simulink model "soccer"  (Simulink 4.00)
settings: Solver=ode45  StartTime=0.0  StopTime=150  RelTol=1e-3
PostLoadFcn:
  | init_motes
InitFcn:
  | clear functions
undefined symbols (not defined in the file or in its folder): WLAN, xBall, xPos, yBall, yPos
libraries: truetime x11
settings Model: Creator=anton  LastModifiedBy=anton  SaveTime=off  SaveOutput=off  RTWOptions="-aEnforceIntegerDowncast=1 -aFoldNonRolledExpr=1 -aInlineInvariantSignals=0 -aInlineParameters=0 -aLocalBlockOutputs=1 -aRollThreshold=5 -aGenerateReport=0 -aGenCodeOnly=0 -aRTWVerbose=1 -aIncludeHyperlinkInReport=0 -aLaunchReport=0 -aForceParamTrailComments=0 -aGenerateComments=1 -aIgnoreCustomStorageClasses=1 -aIncHierarchyInIds=0 -aMaxRTWIdLen=31 -aShowEliminatedStatements=0 -aPrefixModelToSubsysFcnNames=1 -aIncDataTypeInIds=0 -aInsertBlockDesc=0 -aSimulinkBlockComments=1 -aInlinedPrmAccess=\"Literals\"  -aSuppressErrorStatus=0 -aModelReferenceCompliant=1 -aSupportNonInlinedSFcns=1 -aSupportContinuousTime=1 -aSupportComplex=1 -aSupportNonFinite=1 -aSupportAbsoluteTime=1 -aTargetPreCompLibLocation=\"\" -aTargetLibSuffix=\"\" -aTargetFcnLib=\"ansi_tfl_tmw.mat\" -aMultiInstanceERTCode=0 -aLogVarNameModifier=\"rt_\" -aERTFirstTimeCompliant=0 -aIsPILTarget=0 -aCombineOutputUpdateFcns=0 -aGenerateASAP2=0 -aGenerateTestInterfaces=0 -aGenerateSampleERTMain=0 -aGenerateFullHeader=1 -aUtilityFuncGeneration=\"Auto\" -aIncludeFileDelimiter=\"Auto\" -aIncludeERTFirstTime=1 -aIncludeMdlTerminateFcn=1 -aPurelyIntegerCode=0 -aERTCustomFileBanners=0 -aRTWCAPIStates=0 -aRTWCAPIParams=0 -aRTWCAPISignals=0 -aMatFileLogging=1 -aGenFloatMathFcnCalls=\"ANSI_C\" -aExtModeMexFile=\"ext_comm\" -aExtModeTransport=0 -aExtModeStaticAllocSize=1000000 -aExtModeTesting=0 -aExtModeStaticAlloc=0 -aExtMode=0"  ExtModeAutoUpdateStatusClock=off  BlockReductionOpt=off

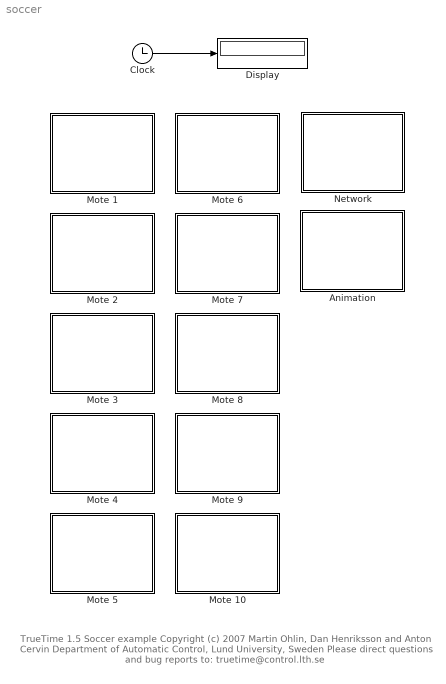
== system soccer ==
  note: TrueTime 1.5  Soccer example
      | Copyright (c) 2007
      | Martin Ohlin, Dan Henriksson and Anton Cervin
      | Department of Automatic Control, Lund University, Sweden
      | Please direct questions and bug reports to:  truetime@control.lth.se
  Animation : Subsystem  mask{N=10}
      mask prompts: N "Number of nodes"
      mask init:
      | %Remove all "From" blocks
      | %Remove all lines from the "From" blocks
      | muxblocks = {'xMux', 'yMux'};
      | fromblocks={'x', 'y'};
      | for j=1:length(muxblocks),
      |   Nold=str2num(get_param(strcat(strcat(gcb,'/'), muxblocks{j}),'Inputs'));
      |   for k=1:Nold
      |     to_name=strcat(strcat(muxblocks{j}, '/'), num2str(k));
      |     from_name=strcat(strcat(fromblocks{j}, num2str(k)), '/1');
      |     delete_line(gcb, from_name, to_name);
      |     delete_block(strcat(strcat(gcb, '/'), strcat(fromblocks{j}, num2str(k))));
      |   end
      |   set_param(strcat(strcat(gcb,'/'), muxblocks{j}),'Inputs',num2str(N));
      | end
      | 
      | for k=1:N
      |     name=strcat(strcat(gcb,'/x'),num2str(k));
      |     add_block('built-in/From',name,'Position',[15 15+(k-1)*20 45 15+k*20],'GotoTag',strcat('x',num2str(k)));
      |     add_line(gcb,strcat(strcat('x',num2str(k)),'/1'),strcat('xMux/',num2str(k)));
      |     
      |     name=strcat(strcat(gcb,'/y'),num2str(k));
      |     add_block('built-in/From',name,'Position',[80 150+(k-1)*20 110 150+k*20],'GotoTag',strcat('y',num2str(k)));
      |     add_line(gcb,strcat(strcat('y',num2str(k)),'/1'),strcat('yMux/',num2str(k)));
      | end
      settings: RTWFcnNameOpts=Auto  RTWFileNameOpts=Auto
  Clock : Clock
      settings: DisplayTime=off  Decimation=10
  Display : Display
      settings: Format=short
  Mote 1 : Subsystem  mask(fgdfgMOTE){nodeID=1}
      mask prompts: nodeID "Node number"
      mask init:
      | set_param(strcat(gcb,'/From_rcv'),'GotoTag',strcat('rcv',num2str(nodeID)));
      | set_param(strcat(gcb,'/Goto_x'),'GotoTag',strcat('x',num2str(nodeID)));
      | set_param(strcat(gcb,'/Goto_y'),'GotoTag',strcat('y',num2str(nodeID)));
      | set_param(strcat(gcb,'/Goto_snd'),'GotoTag',strcat('snd',num2str(nodeID)));
      settings: RTWFcnNameOpts=Auto  RTWFileNameOpts=Auto
  Mote 10 : Subsystem  mask(fgdfgMOTE){nodeID=10}
      mask prompts: nodeID "Node number"
      mask init: same as soccer/Mote 1
      settings: RTWFcnNameOpts=Auto  RTWFileNameOpts=Auto
  Mote 2 : Subsystem  mask(fgdfgMOTE){nodeID=2}
      mask prompts: nodeID "Node number"
      mask init: same as soccer/Mote 1
      settings: RTWFcnNameOpts=Auto  RTWFileNameOpts=Auto
  Mote 3 : Subsystem  mask(fgdfgMOTE){nodeID=3}
      mask prompts: nodeID "Node number"
      mask init: same as soccer/Mote 1
      settings: RTWFcnNameOpts=Auto  RTWFileNameOpts=Auto
  Mote 4 : Subsystem  mask(fgdfgMOTE){nodeID=4}
      mask prompts: nodeID "Node number"
      mask init: same as soccer/Mote 1
      settings: RTWFcnNameOpts=Auto  RTWFileNameOpts=Auto
  Mote 5 : Subsystem  mask(fgdfgMOTE){nodeID=5}
      mask prompts: nodeID "Node number"
      mask init: same as soccer/Mote 1
      settings: RTWFcnNameOpts=Auto  RTWFileNameOpts=Auto
  Mote 6 : Subsystem  mask(fgdfgMOTE){nodeID=6}
      mask prompts: nodeID "Node number"
      mask init: same as soccer/Mote 1
      settings: RTWFcnNameOpts=Auto  RTWFileNameOpts=Auto
  Mote 7 : Subsystem  mask(fgdfgMOTE){nodeID=7}
      mask prompts: nodeID "Node number"
      mask init: same as soccer/Mote 1
      settings: RTWFcnNameOpts=Auto  RTWFileNameOpts=Auto
  Mote 8 : Subsystem  mask(fgdfgMOTE){nodeID=8}
      mask prompts: nodeID "Node number"
      mask init: same as soccer/Mote 1
      settings: RTWFcnNameOpts=Auto  RTWFileNameOpts=Auto
  Mote 9 : Subsystem  mask(fgdfgMOTE){nodeID=9}
      mask prompts: nodeID "Node number"
      mask init: same as soccer/Mote 1
      settings: RTWFcnNameOpts=Auto  RTWFileNameOpts=Auto
  Network : Subsystem  mask{N=10}
      mask prompts: N "Number of nodes"
      mask init:
      | %Remove all "From" blocks
      | %Remove all lines from the "From" blocks
      | muxblocks = {'sndMux', 'xMux', 'yMux'};
      | fromblocks={'snd', 'x', 'y'};
      | for j=1:length(muxblocks),
      |   Nold=str2num(get_param(strcat(strcat(gcb,'/'), muxblocks{j}),'Inputs'));
      |   for k=1:Nold
      |     to_name=strcat(strcat(muxblocks{j}, '/'), num2str(k));
      |     from_name=strcat(strcat(fromblocks{j}, num2str(k)), '/1');
      |     delete_line(gcb, from_name, to_name);
      |     delete_block(strcat(strcat(gcb, '/'), strcat(fromblocks{j}, num2str(k))));
      |   end
      |   set_param(strcat(strcat(gcb,'/'), muxblocks{j}),'Inputs',num2str(N));
      | end
      | 
      | %Remove all "Goto" blocks
      | %Remove all lines to the "Goto" block
      | demuxblocks={'Demux'};
      | gotoblocks={'rcv'};
      | for j=1:length(demuxblocks)
      |   Nold=str2num(get_param(strcat(strcat(gcb,'/'), demuxblocks{j}),'Outputs'));
      |   for k=1:Nold
      |     from_name=strcat(strcat(demuxblocks{j}, '/'), num2str(k));
      |     to_name=strcat(strcat(gotoblocks{j}, num2str(k)), '/1');
      |     delete_line(gcb, from_name, to_name);
      |     delete_block(strcat(strcat(gcb, '/'), strcat(gotoblocks{j}, num2str(k))));
      |   end
      |   set_param(strcat(strcat(gcb, '/'), demuxblocks{j}), 'Outputs',num2str(N));
      | end
      | 
      | 
      | for k=1:N
      |     name=strcat(strcat(gcb,'/snd'),num2str(k));
      |     add_block('built-in/From',name,'Position',[15 30+(k-1)*20 45 30+k*20],'GotoTag',strcat('snd',num2str(k)));
      |     add_line(gcb,strcat(strcat('snd',num2str(k)),'/1'),strcat('sndMux/',num2str(k)));
      |     
      |     name=strcat(strcat(gcb,'/x'),num2str(k));
      |     add_block('built-in/From',name,'Position',[60 130+(k-1)*20 90 130+k*20],'GotoTag',strcat('x',num2str(k)));
      |     add_line(gcb,strcat(strcat('x',num2str(k)),'/1'),strcat('xMux/',num2str(k)));
      |     
      |     name=strcat(strcat(gcb,'/y'),num2str(k));
      |     add_block('built-in/From',name,'Position',[105 230+(k-1)*20 135 230+k*20],'GotoTag',strcat('y',num2str(k)));
      |     add_line(gcb,strcat(strcat('y',num2str(k)),'/1'),strcat('yMux/',num2str(k)));
      | 
      |     name=strcat(strcat(gcb,'/rcv'),num2str(k));
      |     add_block('built-in/Goto',name,'Position',[480 30+(k-1)*20 510 30+k*20],'GotoTag',strcat('rcv',num2str(k)),'TagVisibility','global');
      |     add_line(gcb,strcat('Demux/',num2str(k)),strcat(strcat('rcv',num2str(k)),'/1'));
      | 
      | end
      settings: RTWFcnNameOpts=Auto  RTWFileNameOpts=Auto
  wires:
  Clock/1 -> Display/1

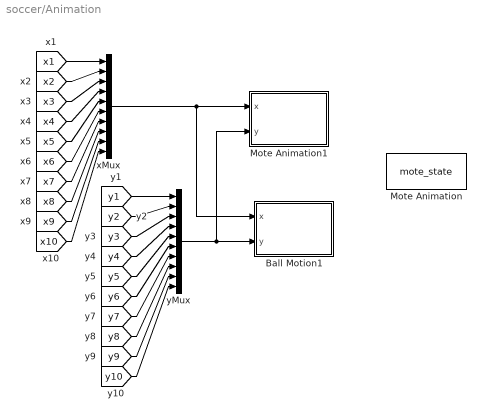
== system soccer/Animation ==
  Ball Motion1 : Subsystem  mask{numMotes=10}
      mask prompts: numMotes "Number of Motes"
      settings: RTWFcnNameOpts=Auto  RTWFileNameOpts=Auto
  Mote Animation : S-Function  FunctionName=mote_state  PortCounts=[]  SFunctionModules=''
      settings: DeleteFcn=if ~isempty(findobj('type','figure','name','dblpend1 Animation'));close('dblpend1 Animation'); end;
  Mote Animation1 : Subsystem  mask{numMotes=10, xmax=20, ymax=30, ts=0.1, x0=xPos, y0=yPos}
      mask prompts: numMotes "Number of Motes"; ts "Update period"
      settings: RTWFcnNameOpts=Auto  RTWFileNameOpts=Auto
  xMux : Mux  Inputs=10
  yMux : Mux  Inputs=10
  wires:
  xMux/1 -> Ball Motion1/1(x), Mote Animation1/1(x)
  yMux/1 -> Mote Animation1/2(y), Ball Motion1/2(y)
  [x1] -> xMux/1
  [y1] -> yMux/1
  [x2] -> xMux/2
  [y2] -> yMux/2
  [x3] -> xMux/3
  [y3] -> yMux/3
  [x4] -> xMux/4
  [y4] -> yMux/4
  [x5] -> xMux/5
  [y5] -> yMux/5
  [x6] -> xMux/6
  [y6] -> yMux/6
  [x7] -> xMux/7
  [y7] -> yMux/7
  [x8] -> xMux/8
  [y8] -> yMux/8
  [x9] -> xMux/9
  [y9] -> yMux/9
  [x10] -> xMux/10
  [y10] -> yMux/10

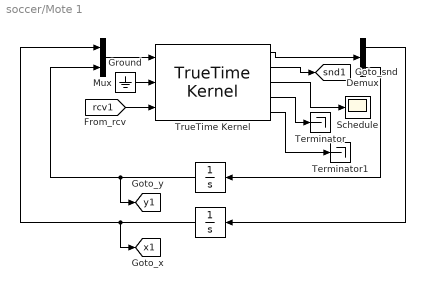
== system soccer/Mote 1 ==
  " " : Integrator  Orientation=left  ExternalReset=none  InitialConditionSource=internal  InitialCondition=yPos(nodeID)  LimitOutput=off  UpperSaturationLimit=inf  LowerSaturationLimit=-inf  ShowSaturationPort=off  ShowStatePort=off  AbsoluteTolerance=auto
  "    " : Integrator  Orientation=left  ExternalReset=none  InitialConditionSource=internal  InitialCondition=xPos(nodeID)  LimitOutput=off  UpperSaturationLimit=inf  LowerSaturationLimit=-inf  ShowSaturationPort=off  ShowStatePort=off  AbsoluteTolerance=auto
  Demux : Demux  Outputs=2  BusSelectionMode=off
  Ground : Ground
  Mux : Mux  Inputs=2
  Schedule : Scope
      settings: TickLabels=on  TimeRange=3.5  YMin=1.8  YMax=3.7  SaveToWorkspace=off  SaveName=ScopeData  DataFormat=Array  MaxDataPoints=5000
  Terminator : Terminator
  Terminator1 : Terminator
  TrueTime Kernel : truetime/TrueTime Kernel  sfun=node_red_goalie_init  args=nodeID  battery=off  clockdrift=0  clockoffset=0
  tag scope: snd1=global, x1=global, y1=global
  wires:
  TrueTime Kernel/3 -> Schedule/1
  Ground/1 -> TrueTime Kernel/2
  [rcv1] -> TrueTime Kernel/3
  Mux/1 -> TrueTime Kernel/1
  TrueTime Kernel/4 -> Terminator/1
  TrueTime Kernel/1 -> Demux/1
  TrueTime Kernel/2 -> [snd1]
  Demux/2 -> " "/1
  Demux/1 -> "    "/1
  " "/1 -> Mux/2, [y1]
  "    "/1 -> Mux/1, [x1]
  TrueTime Kernel/5 -> Terminator1/1

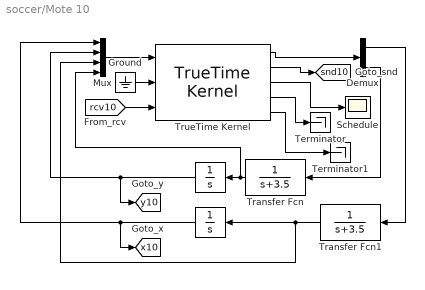
== system soccer/Mote 10 ==
  " " : Integrator  Orientation=left  ExternalReset=none  InitialConditionSource=internal  InitialCondition=yPos(nodeID)  LimitOutput=off  UpperSaturationLimit=inf  LowerSaturationLimit=-inf  ShowSaturationPort=off  ShowStatePort=off  AbsoluteTolerance=auto
  "    " : Integrator  Orientation=left  ExternalReset=none  InitialConditionSource=internal  InitialCondition=xPos(nodeID)  LimitOutput=off  UpperSaturationLimit=inf  LowerSaturationLimit=-inf  ShowSaturationPort=off  ShowStatePort=off  AbsoluteTolerance=auto
  Demux : Demux  Outputs=2  BusSelectionMode=off
  Ground : Ground
  Mux : Mux  Inputs=4
  Schedule : Scope
      settings: TickLabels=on  TimeRange=3.5  YMin=1.8  YMax=3.7  SaveToWorkspace=off  SaveName=ScopeData  DataFormat=Array  MaxDataPoints=5000
  Terminator : Terminator
  Terminator1 : Terminator
  Transfer Fcn : TransferFcn  Orientation=left  Numerator=[1]  Denominator=[1 3.5]  AbsoluteTolerance=auto  Realization=auto
  Transfer Fcn1 : TransferFcn  Orientation=left  Numerator=[1]  Denominator=[1 3.5]  AbsoluteTolerance=auto  Realization=auto
  TrueTime Kernel : truetime/TrueTime Kernel  sfun=node_blue_init  args=nodeID  battery=off  clockdrift=0  clockoffset=0
  tag scope: snd10=global, x10=global, y10=global
  wires:
  TrueTime Kernel/3 -> Schedule/1
  Ground/1 -> TrueTime Kernel/2
  [rcv10] -> TrueTime Kernel/3
  Mux/1 -> TrueTime Kernel/1
  TrueTime Kernel/4 -> Terminator/1
  TrueTime Kernel/1 -> Demux/1
  TrueTime Kernel/2 -> [snd10]
  Demux/2 -> Transfer Fcn/1
  Demux/1 -> Transfer Fcn1/1
  " "/1 -> Mux/2, [y10]
  "    "/1 -> Mux/1, [x10]
  Transfer Fcn/1 -> " "/1, Mux/4
  Transfer Fcn1/1 -> "    "/1, Mux/3
  TrueTime Kernel/5 -> Terminator1/1

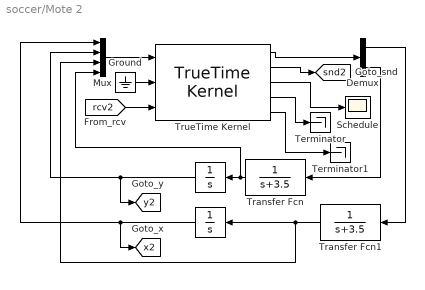
== system soccer/Mote 2 ==
  " " : Integrator  Orientation=left  ExternalReset=none  InitialConditionSource=internal  InitialCondition=yPos(nodeID)  LimitOutput=off  UpperSaturationLimit=inf  LowerSaturationLimit=-inf  ShowSaturationPort=off  ShowStatePort=off  AbsoluteTolerance=auto
  "    " : Integrator  Orientation=left  ExternalReset=none  InitialConditionSource=internal  InitialCondition=xPos(nodeID)  LimitOutput=off  UpperSaturationLimit=inf  LowerSaturationLimit=-inf  ShowSaturationPort=off  ShowStatePort=off  AbsoluteTolerance=auto
  Demux : Demux  Outputs=2  BusSelectionMode=off
  Ground : Ground
  Mux : Mux  Inputs=4
  Schedule : Scope
      settings: TickLabels=on  TimeRange=3.5  YMin=1.8  YMax=3.7  SaveToWorkspace=off  SaveName=ScopeData  DataFormat=Array  MaxDataPoints=5000
  Terminator : Terminator
  Terminator1 : Terminator
  Transfer Fcn : TransferFcn  Orientation=left  Numerator=[1]  Denominator=[1 3.5]  AbsoluteTolerance=auto  Realization=auto
  Transfer Fcn1 : TransferFcn  Orientation=left  Numerator=[1]  Denominator=[1 3.5]  AbsoluteTolerance=auto  Realization=auto
  TrueTime Kernel : truetime/TrueTime Kernel  sfun=node_red_init  args=nodeID  battery=off  clockdrift=0  clockoffset=0
  tag scope: snd2=global, x2=global, y2=global
  wires:
  TrueTime Kernel/3 -> Schedule/1
  Ground/1 -> TrueTime Kernel/2
  [rcv2] -> TrueTime Kernel/3
  Mux/1 -> TrueTime Kernel/1
  TrueTime Kernel/4 -> Terminator/1
  TrueTime Kernel/1 -> Demux/1
  TrueTime Kernel/2 -> [snd2]
  Demux/2 -> Transfer Fcn/1
  Demux/1 -> Transfer Fcn1/1
  " "/1 -> Mux/2, [y2]
  "    "/1 -> Mux/1, [x2]
  Transfer Fcn/1 -> " "/1, Mux/4
  Transfer Fcn1/1 -> "    "/1, Mux/3
  TrueTime Kernel/5 -> Terminator1/1

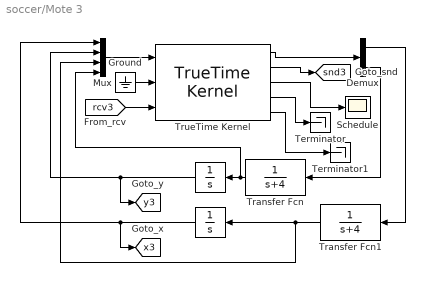
== system soccer/Mote 3 ==
  " " : Integrator  Orientation=left  ExternalReset=none  InitialConditionSource=internal  InitialCondition=yPos(nodeID)  LimitOutput=off  UpperSaturationLimit=inf  LowerSaturationLimit=-inf  ShowSaturationPort=off  ShowStatePort=off  AbsoluteTolerance=auto
  "    " : Integrator  Orientation=left  ExternalReset=none  InitialConditionSource=internal  InitialCondition=xPos(nodeID)  LimitOutput=off  UpperSaturationLimit=inf  LowerSaturationLimit=-inf  ShowSaturationPort=off  ShowStatePort=off  AbsoluteTolerance=auto
  Demux : Demux  Outputs=2  BusSelectionMode=off
  Ground : Ground
  Mux : Mux  Inputs=4
  Schedule : Scope
      settings: TickLabels=on  TimeRange=3.5  YMin=1.8  YMax=3.7  SaveToWorkspace=off  SaveName=ScopeData  DataFormat=Array  MaxDataPoints=5000
  Terminator : Terminator
  Terminator1 : Terminator
  Transfer Fcn : TransferFcn  Orientation=left  Numerator=[1]  Denominator=[1 4]  AbsoluteTolerance=auto  Realization=auto
  Transfer Fcn1 : TransferFcn  Orientation=left  Numerator=[1]  Denominator=[1 4]  AbsoluteTolerance=auto  Realization=auto
  TrueTime Kernel : truetime/TrueTime Kernel  sfun=node_red_init  args=nodeID  battery=off  clockdrift=0  clockoffset=0
  tag scope: snd3=global, x3=global, y3=global
  wires:
  TrueTime Kernel/3 -> Schedule/1
  Ground/1 -> TrueTime Kernel/2
  [rcv3] -> TrueTime Kernel/3
  Mux/1 -> TrueTime Kernel/1
  TrueTime Kernel/4 -> Terminator/1
  TrueTime Kernel/1 -> Demux/1
  TrueTime Kernel/2 -> [snd3]
  Demux/2 -> Transfer Fcn/1
  Demux/1 -> Transfer Fcn1/1
  " "/1 -> Mux/2, [y3]
  "    "/1 -> Mux/1, [x3]
  Transfer Fcn/1 -> " "/1, Mux/4
  Transfer Fcn1/1 -> "    "/1, Mux/3
  TrueTime Kernel/5 -> Terminator1/1

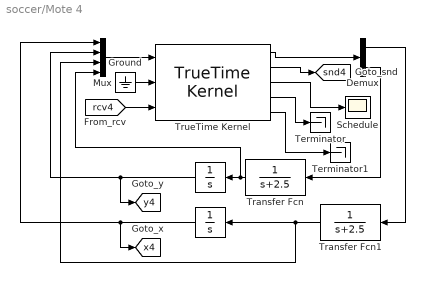
== system soccer/Mote 4 ==
  " " : Integrator  Orientation=left  ExternalReset=none  InitialConditionSource=internal  InitialCondition=yPos(nodeID)  LimitOutput=off  UpperSaturationLimit=inf  LowerSaturationLimit=-inf  ShowSaturationPort=off  ShowStatePort=off  AbsoluteTolerance=auto
  "    " : Integrator  Orientation=left  ExternalReset=none  InitialConditionSource=internal  InitialCondition=xPos(nodeID)  LimitOutput=off  UpperSaturationLimit=inf  LowerSaturationLimit=-inf  ShowSaturationPort=off  ShowStatePort=off  AbsoluteTolerance=auto
  Demux : Demux  Outputs=2  BusSelectionMode=off
  Ground : Ground
  Mux : Mux  Inputs=4
  Schedule : Scope
      settings: TickLabels=on  TimeRange=3.5  YMin=1.8  YMax=3.7  SaveToWorkspace=off  SaveName=ScopeData  DataFormat=Array  MaxDataPoints=5000
  Terminator : Terminator
  Terminator1 : Terminator
  Transfer Fcn : TransferFcn  Orientation=left  Numerator=[1]  Denominator=[1 2.5]  AbsoluteTolerance=auto  Realization=auto
  Transfer Fcn1 : TransferFcn  Orientation=left  Numerator=[1]  Denominator=[1 2.5]  AbsoluteTolerance=auto  Realization=auto
  TrueTime Kernel : truetime/TrueTime Kernel  sfun=node_red_init  args=nodeID  battery=off  clockdrift=0  clockoffset=0
  tag scope: snd4=global, x4=global, y4=global
  wires:
  TrueTime Kernel/3 -> Schedule/1
  Ground/1 -> TrueTime Kernel/2
  [rcv4] -> TrueTime Kernel/3
  Mux/1 -> TrueTime Kernel/1
  TrueTime Kernel/4 -> Terminator/1
  TrueTime Kernel/1 -> Demux/1
  TrueTime Kernel/2 -> [snd4]
  Demux/2 -> Transfer Fcn/1
  Demux/1 -> Transfer Fcn1/1
  " "/1 -> Mux/2, [y4]
  "    "/1 -> Mux/1, [x4]
  Transfer Fcn/1 -> " "/1, Mux/4
  Transfer Fcn1/1 -> "    "/1, Mux/3
  TrueTime Kernel/5 -> Terminator1/1

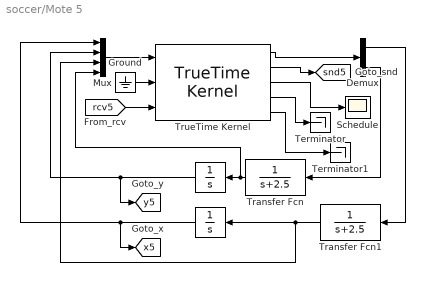
== system soccer/Mote 5 ==
  " " : Integrator  Orientation=left  ExternalReset=none  InitialConditionSource=internal  InitialCondition=yPos(nodeID)  LimitOutput=off  UpperSaturationLimit=inf  LowerSaturationLimit=-inf  ShowSaturationPort=off  ShowStatePort=off  AbsoluteTolerance=auto
  "    " : Integrator  Orientation=left  ExternalReset=none  InitialConditionSource=internal  InitialCondition=xPos(nodeID)  LimitOutput=off  UpperSaturationLimit=inf  LowerSaturationLimit=-inf  ShowSaturationPort=off  ShowStatePort=off  AbsoluteTolerance=auto
  Demux : Demux  Outputs=2  BusSelectionMode=off
  Ground : Ground
  Mux : Mux  Inputs=4
  Schedule : Scope
      settings: TickLabels=on  TimeRange=3.5  YMin=1.8  YMax=3.7  SaveToWorkspace=off  SaveName=ScopeData  DataFormat=Array  MaxDataPoints=5000
  Terminator : Terminator
  Terminator1 : Terminator
  Transfer Fcn : TransferFcn  Orientation=left  Numerator=[1]  Denominator=[1 2.5]  AbsoluteTolerance=auto  Realization=auto
  Transfer Fcn1 : TransferFcn  Orientation=left  Numerator=[1]  Denominator=[1 2.5]  AbsoluteTolerance=auto  Realization=auto
  TrueTime Kernel : truetime/TrueTime Kernel  sfun=node_red_init  args=nodeID  battery=off  clockdrift=0  clockoffset=0
  tag scope: snd5=global, x5=global, y5=global
  wires:
  TrueTime Kernel/3 -> Schedule/1
  Ground/1 -> TrueTime Kernel/2
  [rcv5] -> TrueTime Kernel/3
  Mux/1 -> TrueTime Kernel/1
  TrueTime Kernel/4 -> Terminator/1
  TrueTime Kernel/1 -> Demux/1
  TrueTime Kernel/2 -> [snd5]
  Demux/2 -> Transfer Fcn/1
  Demux/1 -> Transfer Fcn1/1
  " "/1 -> Mux/2, [y5]
  "    "/1 -> Mux/1, [x5]
  Transfer Fcn/1 -> " "/1, Mux/4
  Transfer Fcn1/1 -> "    "/1, Mux/3
  TrueTime Kernel/5 -> Terminator1/1

== system soccer/Mote 6 ==
  " " : Integrator  Orientation=left  ExternalReset=none  InitialConditionSource=internal  InitialCondition=yPos(nodeID)  LimitOutput=off  UpperSaturationLimit=inf  LowerSaturationLimit=-inf  ShowSaturationPort=off  ShowStatePort=off  AbsoluteTolerance=auto
  "    " : Integrator  Orientation=left  ExternalReset=none  InitialConditionSource=internal  InitialCondition=xPos(nodeID)  LimitOutput=off  UpperSaturationLimit=inf  LowerSaturationLimit=-inf  ShowSaturationPort=off  ShowStatePort=off  AbsoluteTolerance=auto
  Demux : Demux  Outputs=2  BusSelectionMode=off
  Ground : Ground
  Mux : Mux  Inputs=2
  Schedule : Scope
      settings: TickLabels=on  TimeRange=3.5  YMin=1.8  YMax=3.7  SaveToWorkspace=off  SaveName=ScopeData  DataFormat=Array  MaxDataPoints=5000
  Terminator : Terminator
  Terminator1 : Terminator
  TrueTime Kernel : truetime/TrueTime Kernel  sfun=node_blue_goalie_init  args=nodeID  battery=off  clockdrift=0  clockoffset=0
  tag scope: snd6=global, x6=global, y6=global
  wires:
  TrueTime Kernel/3 -> Schedule/1
  Ground/1 -> TrueTime Kernel/2
  [rcv6] -> TrueTime Kernel/3
  Mux/1 -> TrueTime Kernel/1
  TrueTime Kernel/4 -> Terminator/1
  TrueTime Kernel/1 -> Demux/1
  TrueTime Kernel/2 -> [snd6]
  Demux/2 -> " "/1
  Demux/1 -> "    "/1
  " "/1 -> Mux/2, [y6]
  "    "/1 -> Mux/1, [x6]
  TrueTime Kernel/5 -> Terminator1/1

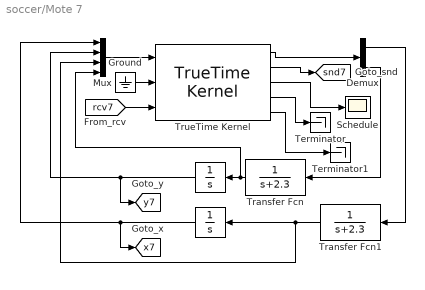
== system soccer/Mote 7 ==
  " " : Integrator  Orientation=left  ExternalReset=none  InitialConditionSource=internal  InitialCondition=yPos(nodeID)  LimitOutput=off  UpperSaturationLimit=inf  LowerSaturationLimit=-inf  ShowSaturationPort=off  ShowStatePort=off  AbsoluteTolerance=auto
  "    " : Integrator  Orientation=left  ExternalReset=none  InitialConditionSource=internal  InitialCondition=xPos(nodeID)  LimitOutput=off  UpperSaturationLimit=inf  LowerSaturationLimit=-inf  ShowSaturationPort=off  ShowStatePort=off  AbsoluteTolerance=auto
  Demux : Demux  Outputs=2  BusSelectionMode=off
  Ground : Ground
  Mux : Mux  Inputs=4
  Schedule : Scope
      settings: TickLabels=on  TimeRange=3.5  YMin=1.8  YMax=3.7  SaveToWorkspace=off  SaveName=ScopeData  DataFormat=Array  MaxDataPoints=5000
  Terminator : Terminator
  Terminator1 : Terminator
  Transfer Fcn : TransferFcn  Orientation=left  Numerator=[1]  Denominator=[1 2.3]  AbsoluteTolerance=auto  Realization=auto
  Transfer Fcn1 : TransferFcn  Orientation=left  Numerator=[1]  Denominator=[1 2.3]  AbsoluteTolerance=auto  Realization=auto
  TrueTime Kernel : truetime/TrueTime Kernel  sfun=node_blue_init  args=nodeID  battery=off  clockdrift=0  clockoffset=0
  tag scope: snd7=global, x7=global, y7=global
  wires:
  TrueTime Kernel/3 -> Schedule/1
  Ground/1 -> TrueTime Kernel/2
  [rcv7] -> TrueTime Kernel/3
  Mux/1 -> TrueTime Kernel/1
  TrueTime Kernel/4 -> Terminator/1
  TrueTime Kernel/1 -> Demux/1
  TrueTime Kernel/2 -> [snd7]
  Demux/2 -> Transfer Fcn/1
  Demux/1 -> Transfer Fcn1/1
  " "/1 -> Mux/2, [y7]
  "    "/1 -> Mux/1, [x7]
  Transfer Fcn/1 -> " "/1, Mux/4
  Transfer Fcn1/1 -> "    "/1, Mux/3
  TrueTime Kernel/5 -> Terminator1/1

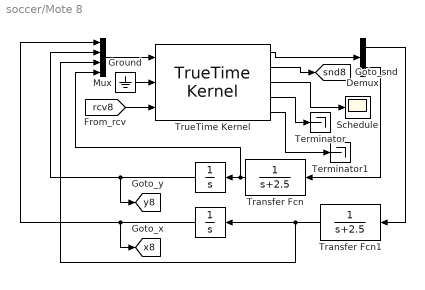
== system soccer/Mote 8 ==
  " " : Integrator  Orientation=left  ExternalReset=none  InitialConditionSource=internal  InitialCondition=yPos(nodeID)  LimitOutput=off  UpperSaturationLimit=inf  LowerSaturationLimit=-inf  ShowSaturationPort=off  ShowStatePort=off  AbsoluteTolerance=auto
  "    " : Integrator  Orientation=left  ExternalReset=none  InitialConditionSource=internal  InitialCondition=xPos(nodeID)  LimitOutput=off  UpperSaturationLimit=inf  LowerSaturationLimit=-inf  ShowSaturationPort=off  ShowStatePort=off  AbsoluteTolerance=auto
  Demux : Demux  Outputs=2  BusSelectionMode=off
  Ground : Ground
  Mux : Mux  Inputs=4
  Schedule : Scope
      settings: TickLabels=on  TimeRange=3.5  YMin=1.8  YMax=3.7  SaveToWorkspace=off  SaveName=ScopeData  DataFormat=Array  MaxDataPoints=5000
  Terminator : Terminator
  Terminator1 : Terminator
  Transfer Fcn : TransferFcn  Orientation=left  Numerator=[1]  Denominator=[1 2.5]  AbsoluteTolerance=auto  Realization=auto
  Transfer Fcn1 : TransferFcn  Orientation=left  Numerator=[1]  Denominator=[1 2.5]  AbsoluteTolerance=auto  Realization=auto
  TrueTime Kernel : truetime/TrueTime Kernel  sfun=node_blue_init  args=nodeID  battery=off  clockdrift=0  clockoffset=0
  tag scope: snd8=global, x8=global, y8=global
  wires:
  TrueTime Kernel/3 -> Schedule/1
  Ground/1 -> TrueTime Kernel/2
  [rcv8] -> TrueTime Kernel/3
  Mux/1 -> TrueTime Kernel/1
  TrueTime Kernel/4 -> Terminator/1
  TrueTime Kernel/1 -> Demux/1
  TrueTime Kernel/2 -> [snd8]
  Demux/2 -> Transfer Fcn/1
  Demux/1 -> Transfer Fcn1/1
  " "/1 -> Mux/2, [y8]
  "    "/1 -> Mux/1, [x8]
  Transfer Fcn/1 -> " "/1, Mux/4
  Transfer Fcn1/1 -> "    "/1, Mux/3
  TrueTime Kernel/5 -> Terminator1/1

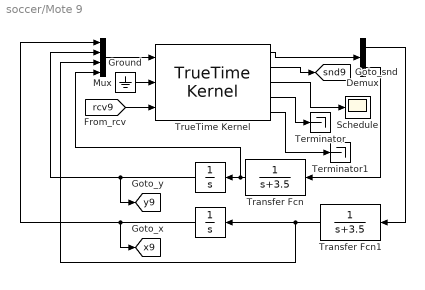
== system soccer/Mote 9 ==
  " " : Integrator  Orientation=left  ExternalReset=none  InitialConditionSource=internal  InitialCondition=yPos(nodeID)  LimitOutput=off  UpperSaturationLimit=inf  LowerSaturationLimit=-inf  ShowSaturationPort=off  ShowStatePort=off  AbsoluteTolerance=auto
  "    " : Integrator  Orientation=left  ExternalReset=none  InitialConditionSource=internal  InitialCondition=xPos(nodeID)  LimitOutput=off  UpperSaturationLimit=inf  LowerSaturationLimit=-inf  ShowSaturationPort=off  ShowStatePort=off  AbsoluteTolerance=auto
  Demux : Demux  Outputs=2  BusSelectionMode=off
  Ground : Ground
  Mux : Mux  Inputs=4
  Schedule : Scope
      settings: TickLabels=on  TimeRange=3.5  YMin=1.8  YMax=3.7  SaveToWorkspace=off  SaveName=ScopeData  DataFormat=Array  MaxDataPoints=5000
  Terminator : Terminator
  Terminator1 : Terminator
  Transfer Fcn : TransferFcn  Orientation=left  Numerator=[1]  Denominator=[1 3.5]  AbsoluteTolerance=auto  Realization=auto
  Transfer Fcn1 : TransferFcn  Orientation=left  Numerator=[1]  Denominator=[1 3.5]  AbsoluteTolerance=auto  Realization=auto
  TrueTime Kernel : truetime/TrueTime Kernel  sfun=node_blue_init  args=nodeID  battery=off  clockdrift=0  clockoffset=0
  tag scope: snd9=global, x9=global, y9=global
  wires:
  TrueTime Kernel/3 -> Schedule/1
  Ground/1 -> TrueTime Kernel/2
  [rcv9] -> TrueTime Kernel/3
  Mux/1 -> TrueTime Kernel/1
  TrueTime Kernel/4 -> Terminator/1
  TrueTime Kernel/1 -> Demux/1
  TrueTime Kernel/2 -> [snd9]
  Demux/2 -> Transfer Fcn/1
  Demux/1 -> Transfer Fcn1/1
  " "/1 -> Mux/2, [y9]
  "    "/1 -> Mux/1, [x9]
  Transfer Fcn/1 -> " "/1, Mux/4
  Transfer Fcn1/1 -> "    "/1, Mux/3
  TrueTime Kernel/5 -> Terminator1/1

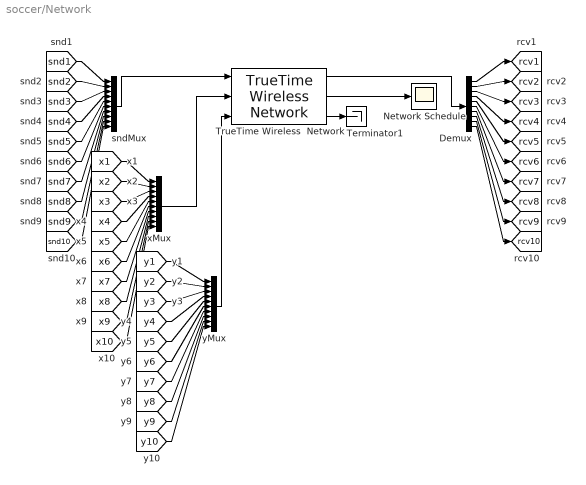
== system soccer/Network ==
  Demux : Demux  Outputs=10  BusSelectionMode=off
  Network Schedule : Scope
      settings: TimeRange=40  YMin=1  YMax=3.5  SaveToWorkspace=off  SaveName=nschedule  MaxDataPoints=5000
  Terminator1 : Terminator
  TrueTime Wireless  Network : truetime/TrueTime Wireless  Network  nwtype=802.11b (WLAN)  nwnbr=1  nnodes=N  rate=800000  minsize=272  transpower=20  threshold=-48  pathloss=3.5  use_pathloss_function=off  acktimeout=0.00004  retrylimit=5  error_threshold=0.03
  sndMux : Mux  Inputs=10
  xMux : Mux  Inputs=10
  yMux : Mux  Inputs=10
  tag scope: rcv10=global, rcv1=global, rcv2=global, rcv3=global, rcv4=global, rcv5=global, rcv6=global, rcv7=global, rcv8=global, rcv9=global
  wires:
  TrueTime Wireless  Network/3 -> Terminator1/1
  sndMux/1 -> TrueTime Wireless  Network/1
  TrueTime Wireless  Network/1 -> Demux/1
  xMux/1 -> TrueTime Wireless  Network/2
  TrueTime Wireless  Network/2 -> Network Schedule/1
  yMux/1 -> TrueTime Wireless  Network/3
  [snd1] -> sndMux/1
  [x1] -> xMux/1
  [y1] -> yMux/1
  Demux/1 -> [rcv1]
  [snd2] -> sndMux/2
  [x2] -> xMux/2
  [y2] -> yMux/2
  Demux/2 -> [rcv2]
  [snd3] -> sndMux/3
  [x3] -> xMux/3
  [y3] -> yMux/3
  Demux/3 -> [rcv3]
  [snd4] -> sndMux/4
  [x4] -> xMux/4
  [y4] -> yMux/4
  Demux/4 -> [rcv4]
  [snd5] -> sndMux/5
  [x5] -> xMux/5
  [y5] -> yMux/5
  Demux/5 -> [rcv5]
  [snd6] -> sndMux/6
  [x6] -> xMux/6
  [y6] -> yMux/6
  Demux/6 -> [rcv6]
  [snd7] -> sndMux/7
  [x7] -> xMux/7
  [y7] -> yMux/7
  Demux/7 -> [rcv7]
  [snd8] -> sndMux/8
  [x8] -> xMux/8
  [y8] -> yMux/8
  Demux/8 -> [rcv8]
  [snd9] -> sndMux/9
  [x9] -> xMux/9
  [y9] -> yMux/9
  Demux/9 -> [rcv9]
  [snd10] -> sndMux/10
  [x10] -> xMux/10
  [y10] -> yMux/10
  Demux/10 -> [rcv10]

== system soccer/Animation/Ball Motion1 ==
  x : Inport  Port=1  LatchInput=off
  y : Inport  Port=2  LatchInput=off
  Mote Animation : S-Function  FunctionName=ballmotion  Parameters=[numMotes,xBall,yBall]  PortCounts=[]  SFunctionModules=''
      settings: DeleteFcn=if ~isempty(findobj('type','figure','name','dblpend1 Animation'));close('dblpend1 Animation'); end;
  Mux : Mux  Inputs=2
  wires:
  x/1 -> Mux/1
  y/1 -> Mux/2
  Mux/1 -> Mote Animation/1

== system soccer/Animation/Mote Animation1 ==
  x : Inport  Port=1  LatchInput=off
  y : Inport  Port=2  LatchInput=off
  Mote Animation : S-Function  FunctionName=moteanimation  Parameters=[numMotes ts xmax ymax] x0 y0  PortCounts=[]  SFunctionModules=''
      settings: DeleteFcn=if ~isempty(findobj('type','figure','name','dblpend1 Animation'));close('dblpend1 Animation'); end;
  Mux : Mux  Inputs=2
  wires:
  Mux/1 -> Mote Animation/1
  y/1 -> Mux/2
  x/1 -> Mux/1
